simulink model "Wired_BER"  (R2018b)
settings: Solver=ode45  StartTime=0.0  StopTime=0  RelTol=1e-3  EnableMultiTasking=on
libraries: commrandsrc2 x1, commsink2 x1
settings Model: Creator=divyang  LastModifiedBy=DSP_06
settings DataIOCC: LimitDataPoints=on  SaveFormat=Array  SignalLoggingSaveFormat=ModelDataLogs
settings OptimizationCC: ExpressionDepthLimit=2147483647  InitFltsAndDblsToZero=on  LifeSpan=inf
settings DebuggingCC: UnderspecifiedInitializationDetection=Classic  MergeDetectMultiDrivingBlocksExec=none  SolverPrmCheckMsg=warning  FcnCallInpInsideContextMsg=warning  AllowSymbolicDim=off  StateNameClashWarn=warning  SFUnexpectedBacktrackingDiag=warning  SFNoUnconditionalDefaultTransitionDiag=warning  SFExecutionAtInitializationDiag=none
settings HardwareCC: ProdBitPerPointer=32  ProdBitPerSizeT=32  ProdBitPerPtrDiffT=32  ProdLargestAtomicFloat=None  ProdIntDivRoundTo=Undefined  ProdEndianess=Unspecified  ProdWordSize=32  ProdHWDeviceType=32-bit Generic
settings ModelReferenceCC: PropagateSignalLabelsOutOfModel=off
settings SFSimCC: SimUseLocalCustomCode=off  SimParseCustomCode=off
settings RTWCC: RTWUseLocalCustomCode=off
settings CodeAppCC: StateflowObjectComments=on
settings GRTTargetCC: TargetLangStandard=C89/C90 (ANSI)  CombineOutputUpdateFcns=off  GRTInterface=on
settings ConfigComp: CovMetricSettings=dw  CovHtmlReporting=on  CovSaveCumulativeToWorkspaceVar=on  CovSaveSingleToWorkspaceVar=on  CovExternalEMLEnable=off

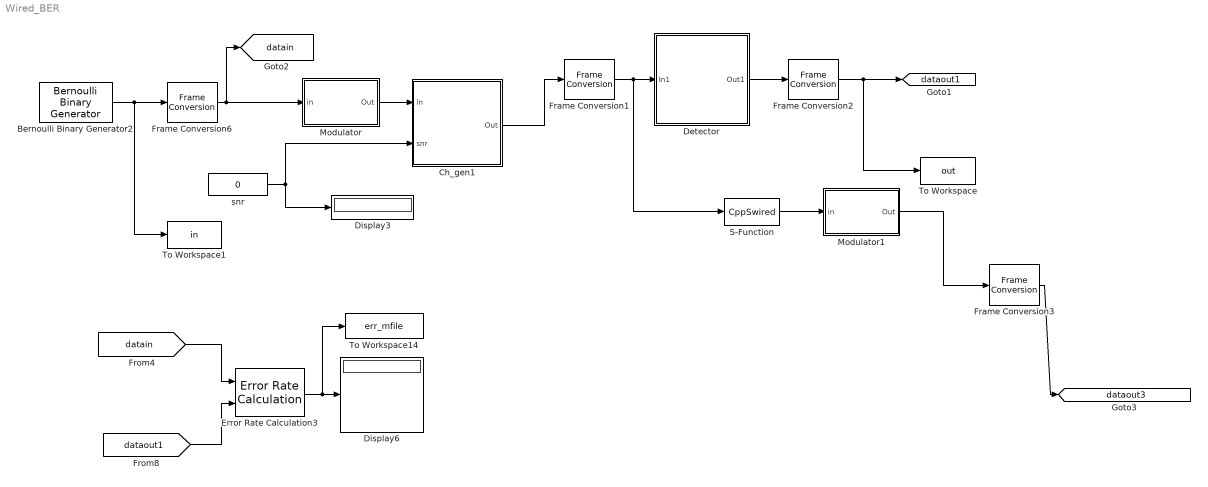
== system Wired_BER ==
  Bernoulli Binary Generator2 : commrandsrc2/Bernoulli Binary Generator  P=0.5  seed=randi(2,1)  Ts=1/(2*14208)  frameBased=on  sampPerFrame=2*14208  orient=off  outDataType=double
  Ch_gen1 : MATLAB Function  TreatAsAtomicUnit=on
  Detector : Subsystem
  Display3 : Display
  Display6 : Display
  Error Rate Calculation3 : commsink2/Error Rate Calculation  N=0  st_delay=0  cp_mode=Entire frame  subframe=[]  PMode=Port  WsName=ErrorVec  RsMode2=off  stop=off  numErr=100  maxBits=1e6
  Frame Conversion{1..3,6} (4 alike) : FrameConversion
  Modulator : MATLAB Function  TreatAsAtomicUnit=on
  Modulator1 : MATLAB Function  TreatAsAtomicUnit=on
  S-Function : S-Function  FunctionName=CppSwired  Parameters=inlen1  SFunctionDeploymentMode=off  EnableBusSupport=off  mask{inlen1=14208/2}
      mask prompts: inlen1 "inplen1"
  To Workspace : ToWorkspace  VariableName=out  SampleTime=-1
      settings: Save2DSignal=2-D array (concatenate along first dimension)
  To Workspace1 : ToWorkspace  VariableName=in  SampleTime=-1
      settings: Save2DSignal=2-D array (concatenate along first dimension)
  To Workspace14 : ToWorkspace  VariableName=err_mfile  SampleTime=-1
  snr : Constant  Value=0
  tag scope: datain=global, dataout1=global, dataout3=global
  wires:
  [datain] -> Error Rate Calculation3/1
  [dataout1] -> Error Rate Calculation3/2
  Error Rate Calculation3/1 -> To Workspace14/1, Display6/1
  S-Function/1 -> Modulator1/1(in)
  snr/1 -> Ch_gen1/2(snr), Display3/1
  Frame Conversion6/1 -> [datain], Modulator/1(in)
  Bernoulli Binary Generator2/1 -> To Workspace1/1, Frame Conversion6/1
  Detector/1(Out1) -> Frame Conversion2/1
  Ch_gen1/1(Out) -> Frame Conversion1/1
  Frame Conversion2/1 -> To Workspace/1, [dataout1]
  Modulator/1(Out) -> Ch_gen1/1(in)
  Frame Conversion1/1 -> S-Function/1, Detector/1(In1)
  Modulator1/1(Out) -> Frame Conversion3/1
  Frame Conversion3/1 -> [dataout3]

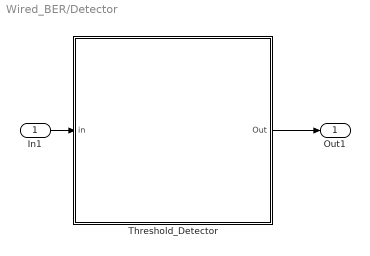
== system Wired_BER/Detector ==
  In1 : Inport
  Threshold_Detector : MATLAB Function  TreatAsAtomicUnit=on
  Out1 : Outport
  wires:
  In1/1 -> Threshold_Detector/1(in)
  Threshold_Detector/1(Out) -> Out1/1

== matlab function Wired_BER/Modulator ==
  data: in input; Out output
function Out = mod(in)
[M,N] = size(in);
%Out1 = zeros(M,1);
Out = zeros(M/2,1);
j=1;
for i =1:2:M
    if(in(i) == 0&&in(i+1)==0)
        Out(j) = 1+(1*i);
    end
    if(in(i) == 0&&in(i+1)==1)
        Out(j) = -1+1*i;
    end
    if(in(i) == 1&&in(i+1)==0)
        Out(j) = -1-1*i;
    end
    if(in(i) == 1&&in(i+1)==1)
        Out(j) = 1-1*i;
    end
    j=j+1;
end

== matlab function Wired_BER/Modulator1 ==
  data: in input; Out output
function Out = mod(in)
Out = real(in);

== matlab function Wired_BER/Detector/Threshold_Detector ==
  data: Out output; in input
function Out = Detector(in)
k = 1;
[M,N] =size(in);
out=zeros(2*M,1);

for i=1:M
    
    if(real(in(i)) >0 && imag(in(i)) >0)
        out(k) = 1;
        out(k+1)=1;
    end

    if(real(in(i)) <0 && imag(in(i)) >0)
        out(k) = -1;
        out(k+1)=1;
    end
    
if(real(in(i)) >0 && imag(in(i)) <0)
        out(k) = 1;
        out(k+1)=-1;
end
    
if(real(in(i)) <0 && imag(in(i)) <0)
        out(k) = -1;
        out(k+1)=-1;
end

    
k = k+2;
end
Out = double(out);

== matlab function Wired_BER/Ch_gen1 ==
  data: in input; Out output; snr input
function Out = ch(in,snr)
[M,N] = size(in);
Out = zeros(M,1);
n_var = 1/(10^(snr/10));

Out =  in + ((n_var/2)^0.5)*(randn(M,1));
